simulink model "LKAS"  (R2018b)
settings: Solver=FixedStepDiscrete  StartTime=0.0  StopTime=10.0  FixedStep=0.01  RelTol=1e-3
InitFcn:
  | tmpVer = ver('MATLAB');
  | tmpVer = str2num(tmpVer.Version);
  | % -------------------------------------------------------------------
  | %  MATLAB file generated by Simulink.saveVars on 21-Nov-2019 10:06:14
  | %  MATLAB version: 7.13.0.564 (R2011b)
  | % -------------------------------------------------------------------
  | 
  | 
  | SInt16 = Simulink.AliasType;
  | SInt16.Description = 'Num';
  | if (tmpVer > 7.11)
  | 	SInt16.DataScope = 'Auto';
  | end
  | SInt16.HeaderFile = 'Rte_Type.h';
  | SInt16.BaseType = 'int16';
  | 
  | SInt32 = Simulink.AliasType;
  | SInt32.Description = 'Num';
  | if (tmpVer > 7.11)
  | 	SInt32.DataScope = 'Auto';
  | end
  | SInt32.HeaderFile = 'Rte_Type.h';
  | SInt32.BaseType = 'int32';
  | 
  | SInt8 = Simulink.AliasType;
  | SInt8.Description = 'Num';
  | if (tmpVer > 7.11)
  | 	SInt8.DataScope = 'Auto';
  | end
  | SInt8.HeaderFile = 'Rte_Type.h';
  | SInt8.BaseType = 'int8';
  | 
  | T_A_m2_1024_1_u32 = Simulink.NumericType;
  | T_A_m2_1024_1_u32.Description = 'm2 (square meters  (m2))';
  | if (tmpVer > 7.11)
  | 	T_A_m2_1024_1_u32.DataScope = 'Auto';
  | end
  | T_A_m2_1024_1_u32.HeaderFile = 'Rte_Type.h';
  | T_A_m2_1024_1_u32.DataTypeMode = 'Fixed-point: slope and bias scaling';
  | T_A_m2_1024_1_u32.SignednessBool = false;
  | T_A_m2_1024_1_u32.WordLength = 32;
  | T_A_m2_1024_1_u32.FixedExponent = -10;
  | T_A_m2_1024_1_u32.SlopeAdjustmentFactor = 1;
  | T_A_m2_1024_1_u32.Bias = 0;
  | T_A_m2_1024_1_u32.DataTypeOverride = 'Inherit';
  | T_A_m2_1024_1_u32.IsAlias = true;
  | 
  | T_A_m2_65536_1_u16 = Simulink.NumericType;
  | T_A_m2_65536_1_u16.Description = 'm2 (square meters  (m2))';
  | if (tmpVer > 7.11)
  | 	T_A_m2_65536_1_u16.DataScope = 'Auto';
  | end
  | T_A_m2_65536_1_u16.HeaderFile = 'Rte_Type.h';
  | T_A_m2_65536_1_u16.DataTypeMode = 'Fixed-point: slope and bias scaling';
  | T_A_m2_65536_1_u16.SignednessBool = false;
  | T_A_m2_65536_1_u16.WordLength = 16;
  | T_A_m2_65536_1_u16.FixedExponent = -16;
  | T_A_m2_65536_1_u16.SlopeAdjustmentFactor = 1;
  | T_A_m2_65536_1_u16.Bias = 0;
  | T_A_m2_65536_1_u16.DataTypeOverride = 'Inherit';
  | ... (+4598 lines)
StopFcn:
  | clear  T_A_m2_1024_1_u32 T_A_m2_65536_1_u16 T_A_m2_Float32 T_A_mm2_10_1_u16 T_A_mm2_4_1_s16 T_A_mm2_Float32 T_Cnt_Num_10_1_u32 T_Cnt_Num_1_1_s16 T_Cnt_Num_1_1_s32 T_Cnt_Num_1_1_s8 T_Cnt_Num_1_1_u16 T_Cnt_Num_1_1_u32 T_Cnt_Num_1_1_u8 T_E_J_1_1_s32 T_E_J_Float32 T_E_kJ_128_1_s32 T_E_kJ_Float32 T_E_kwh_10_1_u16 T_E_kwh_Float32 T_Epl_kwhpkm_100_1_u16 T_Epl_kwhpkm_Float32 T_F_N_1_1_s16 T_F_N_Float32 T_I_A_1000_1_u16 T_I_A_1048576_1_s32 T_I_A_2048_1_s16 T_I_A_32_1_s16 T_I_A_Float32 T_I_mA_1_1_s16 T_I_mA_32768_128_s16 T_I_mA_Float32 T_J_kgpm2_128_1_u16 T_J_kgpm2_Float32 T_K_NA_1000_1_s16 T_K_NA_100_1_s16 T_K_NA_100_1_u16 T_K_NA_1024_1_s16 T_K_NA_1024_1_u16 T_K_NA_128_1_s16 T_K_NA_128_1_u16 T_K_NA_128_1_u8 T_K_NA_16777216_1_u32 T_K_NA_16_1_s16 T_K_NA_16_1_u16 T_K_NA_16_1_u8 T_K_NA_1_16_u16 T_K_NA_1_1_s16 T_K_NA_1_1_u16 T_K_NA_1_1_u8 T_K_NA_32768_1_s16 T_K_NA_32768_1_u16 T_K_NA_32_1_s8 T_K_NA_4096_1_u16 T_K_NA_4194304_1_s32 T_K_NA_4194304_1_u16 T_K_NA_65536_1_s32 T_K_NA_65536_1_u16 T_K_NA_8192_1_s16 T_K_NA_8_1_s16 T_K_NA_Float32 T_M_Nm_16_1_s16 T_M_Nm_1_1_s16 T_M_Nm_32768_1_s16 T_M_Nm_32_1_s16 T_M_Nm_4_1_s16 T_M_Nm_512_1_s16 T_M_Nm_Float32 T_P_W_1_4_s16 T_P_W_1_8_s16 T_P_W_Float32 T_P_kW_128_1_s16 T_P_kW_1_8_s16 T_P_kW_8_1_s32 T_P_kW_Float32 T_Pct_pct_1024_1_s32 T_Pct_pct_1024_1_u32 T_Pct_pct_10_1_s16 T_Pct_pct_10_1_u32 T_Pct_pct_128_100_s8 T_Pct_pct_1_1_s16 T_Pct_pct_1_4_u8 T_Pct_pct_255_100_u16 T_Pct_pct_255_100_u8 T_Pct_pct_256_1_s16 T_Pct_pct_256_1_u16 T_Pct_pct_65535_100_u16 T_Pct_pct_Float32 T_R_ohm_1024_1_s16 T_R_ohm_32_1_s16 T_R_ohm_Float32 T_TK_K_16_1_s16 T_TK_K_Float32 T_T_degC_10_400_1_u16 T_T_degC_16_1_s16 T_T_degC_1_40_1_u8 T_T_degC_2_80_1_u8 T_T_degC_Float32 T_U_V_1000_1_u16 T_U_V_10_1_u8 T_U_V_200_1_u8 T_U_V_32_1_s16 T_U_V_4096_1_s16 T_U_V_512_1_s16 T_U_V_65535_8_u16 T_U_V_8192_1_u16 T_U_V_Float32 T_U_mV_1_1_s16 T_U_mV_256_20_u16 T_U_mV_Float32 T_V_l_256_1_s16 T_V_l_4096_1_s16 T_V_l_64_1_s16 T_V_l_65535_100_u16 T_V_l_Float32 T_V_ml_128_1_s16 T_V_ml_1_1_s16 T_V_ml_32768_1_s16 T_V_ml_Float32 T_V_ul_32_1_u16 T_V_ul_Float32 T_Vpl_clpkm_512_1_u16 T_Vpl_clpkm_Float32 T_a_kphps_16_1_s16 T_a_kphps_Float32 T_a_mps2_128_1_s16 T_a_mps2_Float32 T_c_MJpkg_256_1_s16 T_c_MJpkg_Float32 T_c_kJpgpK_1024_1_s16 T_c_kJpgpK_Float32 T_c_kJpkgpK_128_1_u16 T_c_kJpkgpK_Float32 T_chrg_Ah_1_1_s16 T_chrg_Ah_1_1_u16 T_chrg_Ah_1_1_u8 T_chrg_Ah_256_1_u16 T_chrg_Ah_4194304_1_s32 T_chrg_Ah_512_1_u16 T_chrg_Ah_8_1_u16 T_chrg_Ah_Float32 T_cmp_NA_100_1_s16 T_cmp_NA_128_1_s16 T_cmp_NA_16_1_s16 T_cmp_NA_32768_1_u16 T_cmp_NA_Float32 T_d2n_rpmps2_4_1_s16 T_d2n_rpmps2_Float32 T_dPct_pctps_16_1_s16 T_dPct_pctps_256_1_s16 T_dPct_pctps_Float32 T_dT_degCps_128_1_s16 T_dT_degCps_Float32 T_dV_lph_1_1_s16 T_dV_lph_Float32 T_dV_lpm_128_1_s16 T_dV_lpm_32_1_s16 T_dV_lpm_Float32 T_dV_lps_1024_1_u16 T_dV_lps_4_1_u16 T_dV_lps_Float32 T_dV_mlps_1024_1_s16 T_dV_mlps_Float32 T_d_BitField16 T_dm_gps_128_1_s16 T_dm_gps_128_1_u16 T_dm_gps_256_1_u16 T_dm_gps_Float32 T_dm_mgps_1_1_s16 T_dm_mgps_Float32 T_dn_rpmps_1_1_s16 T_dn_rpmps_2_1_s16 T_dn_rpmps_Float32 T_dp_Paps_1_1_s16 T_dp_Paps_Float32 T_dp_kPaps_1_1_s16 T_dp_kPaps_8_1_s16 T_dp_kPaps_Float32 T_dphi_degps_128_1_s16 T_dphi_degps_8_1_s16 T_dphi_degps_Float32 T_dr_ps_256_1_s16 T_dr_ps_Float32 T_drho_mgplps_1_2_s16 T_drho_mgplps_Float32 T_e_NA_1_1_u8 T_f_Hz_1_1_u16 T_f_Hz_1_1_u32 T_f_Hz_64_1_u16 T_f_Hz_8_1_s16 T_f_Hz_Float32 T_g_BitField32 T_l_km_16_1_s16 T_l_km_1_1_u16 T_l_km_1_1_u32 T_l_km_Float32 T_l_m_1024_1_s16 T_l_m_16_1_s16 T_l_m_1_1_u32 T_l_m_Float32 T_l_mm_16_1_s16 T_l_mm_1_1_u16 T_l_mm_4096_1_s16 T_l_mm_4_1_u8 T_l_mm_64_1_s16 T_l_mm_Float32 T_m_g_1_1_s16 T_m_g_2048_1_s16 T_m_g_32_1_u16 T_m_g_Float32 T_m_kg_1024_1_s16 T_m_kg_1_1_s16 T_m_kg_1_1_u32 T_m_kg_Float32 T_m_mg_128_1_s16 T_m_mg_32_1_s16 T_m_mg_Float32 T_n_rpm_1_1_s16 T_n_rpm_1_25_u8 T_n_rpm_256_50_u16 T_n_rpm_2_25_u8 T_n_rpm_4_1_u16 T_n_rpm_Float32 T_p_MPa_64_1_s16 T_p_MPa_Float32 T_p_Pa_1_1_s16 T_p_Pa_Float32 T_p_kPa_1_10_u16 T_p_kPa_1_1_s16 T_p_kPa_1_1_u8 T_p_kPa_256_1_u16 T_p_kPa_32_1_u16 T_p_kPa_64_1_s16 T_p_kPa_Float32 T_phi_deg_100_1_s16 T_phi_deg_1024_1_s16 T_phi_deg_128_1_s16 T_phi_deg_1_1_u8 T_phi_deg_256_1_s16 T_phi_deg_2_1_s8 T_phi_deg_32_1_s16 T_phi_deg_512_6_s32 T_phi_deg_Float32 T_phi_rad_2048_1_s16 T_phi_rad_Float32 T_r_NA_1024_1_s16 T_r_NA_1024_1_u16 T_r_NA_16384_1_s16 T_r_NA_16_1_s16 T_r_NA_256_1_s8 T_r_NA_256_1_u16 T_r_NA_32768_1_u16 T_r_NA_32_1_u16 T_r_NA_4096_1_s16 T_r_NA_65535_2_u16 T_r_NA_8192_1_u16 T_r_NA_Float32 T_rho_gpl_8192_1_s16 T_rho_gpl_Float32 T_rho_kgpm3_16_1_s16 T_rho_kgpm3_Float32 T_rho_mgpl_1_1_s16 T_rho_mgpl_64_1_s16 T_rho_mgpl_Float32 T_t_hour_1_1_s16 T_t_hour_Float32 T_t_m_1_1_u16 T_t_m_Float32 T_t_ms_1_1_s16 T_t_ms_1_1_u16 T_t_ms_1_1_u32 T_t_ms_4096_1_s16 T_t_ms_64_1_s16 T_t_ms_Float32 T_t_s_1000_1_s16 T_t_s_100_1_s16 T_t_s_10_1_s16 T_t_s_10_1_u16 T_t_s_1_1_s16 T_t_s_1_1_u16 T_t_s_1_1_u32 T_t_s_Float32 T_t_us_10_1_u32 T_t_us_1_1_s16 T_t_us_1_1_u32 T_t_us_1_4_u16 T_t_us_Float32 T_v_kph_1_1_u8 T_v_kph_64_1_s16 T_v_kph_64_1_u16 T_v_kph_Float32 T_v_mps_256_1_s16 T_v_mps_Float32 T_w_radps_32_1_s16 T_w_radps_Float32 T_y_BitField8 T_y_BitFieldDiagProgress T_y_BitFieldDiagStatus T_y_NA_1_1_u8 SInt16 SInt32 SInt8 T_BOOLEAN UInt16 UInt32 UInt8 s16 s32 s8 u16 u32 u8
model workspace (MAT data in the model file):
  MCOS : class17 (value not decoded)
  MCOS : class17 (value not decoded)
  MCOS : class17 (value not decoded)
  MCOS : class17 (value not decoded)
  MCOS : class17 (value not decoded)
  MCOS : class17 (value not decoded)
  MCOS : class17 (value not decoded)
  MCOS : class17 (value not decoded)
  MCOS : class17 (value not decoded)
  MCOS : class17 (value not decoded)
  MCOS : class17 (value not decoded)
  MCOS : class17 (value not decoded)
  MCOS : class17 (value not decoded)
  MCOS : class17 (value not decoded)
  MCOS : class17 (value not decoded)
  MCOS : class17 (value not decoded)
  MCOS : class17 (value not decoded)
  MCOS : class17 (value not decoded)
  MCOS : class17 (value not decoded)
  MCOS : class17 (value not decoded)
  MCOS : class17 (value not decoded)
  MCOS : class17 (value not decoded)
  MCOS : class17 (value not decoded)
  MCOS : class17 (value not decoded)
  MCOS : class17 (value not decoded)
  MCOS : class17 (value not decoded)
  MCOS : class17 (value not decoded)
  MCOS : class17 (value not decoded)
  MCOS : class17 (value not decoded)
  MCOS : class17 (value not decoded)
  MCOS : class17 (value not decoded)
  MCOS : class17 (value not decoded)
  MCOS : class17 (value not decoded)
  MCOS : class17 (value not decoded)
  MCOS : class17 (value not decoded)
  MCOS : class17 (value not decoded)
  MCOS : class17 (value not decoded)
  MCOS : class17 (value not decoded)
  MCOS : class17 (value not decoded)
  MCOS : class17 (value not decoded)
  MCOS : class17 (value not decoded)
  MCOS : class17 (value not decoded)
  MCOS : class17 (value not decoded)
  MCOS : class17 (value not decoded)
  MCOS : class17 (value not decoded)
  MCOS : class17 (value not decoded)
  MCOS : class17 (value not decoded)
  MCOS : class17 (value not decoded)
  MCOS : class17 (value not decoded)
  MCOS : class17 (value not decoded)
  MCOS : class17 (value not decoded)
  MCOS : class17 (value not decoded)
  MCOS : class17 (value not decoded)
  MCOS : class17 (value not decoded)
  MCOS : class17 (value not decoded)
  MCOS : class17 (value not decoded)
  MCOS : class17 (value not decoded)
  MCOS : class17 (value not decoded)
  MCOS : class17 (value not decoded)
  MCOS : class17 (value not decoded)
  MCOS : class17 (value not decoded)
  MCOS : class17 (value not decoded)
  MCOS : class17 (value not decoded)
  MCOS : class17 (value not decoded)
  MCOS : class17 (value not decoded)
  MCOS : class17 (value not decoded)
  MCOS : class17 (value not decoded)
  MCOS : class17 (value not decoded)
  MCOS : class17 (value not decoded)
  MCOS : class17 (value not decoded)
  MCOS : class17 (value not decoded)
  MCOS : class17 (value not decoded)
  MCOS : class17 (value not decoded)
  MCOS : class17 (value not decoded)
  MCOS : class17 (value not decoded)
  MCOS : class17 (value not decoded)
  MCOS : class17 (value not decoded)
  MCOS : class17 (value not decoded)
  MCOS : class17 (value not decoded)
  MCOS : class17 (value not decoded)
  MCOS : class17 (value not decoded)
  MCOS : class17 (value not decoded)
  MCOS : class17 (value not decoded)
  MCOS : class17 (value not decoded)
  MCOS : class17 (value not decoded)
  MCOS : class17 (value not decoded)
  MCOS : class17 (value not decoded)
  MCOS : class17 (value not decoded)
  MCOS : class17 (value not decoded)
undefined symbols (not defined in the file): LKA_CarWidth, LKA_SampleTime, LKA_StrRatio_C, LKA_Veh2CamL_C, LKA_Veh2CamW_C, LKA_WhlBaseL_C, LL_CompSWA_C, LL_CrvtPrvwT_C, LL_DesDvt_C, LL_DvtComp_C, LL_DvtPrvwT_C, LL_DvtSpdDet_vDvtSpdMin_C, LL_HdAgExT_C, LL_HdAgPrvwT_C, LL_LAccMax_C, LL_LAccRMax_C, LL_LDW_EarliestWarnLine_C, LL_LDW_LatestWarnLine_C, LL_LDWS_SUPPRESS_HEADING, LL_LFClb_TFC_DiffCtlBalance, LL_LFClb_TFC_DiffCtrlMaxSWA, LL_LFClb_TFC_DiffCtrlRatio, LL_LFClb_TFC_facmGainLutGain1_C, LL_LFClb_TFC_facmGainLutGain2_C, LL_LFClb_TFC_facmIntegRatio, LL_LFClb_TFC_facmKlat_C, LL_LFClb_TFC_FfCtlRatio_C, LL_LFClb_TFC_phiIntegCtlMaxSWA_C, LL_LFClb_TFC_tiKlatPrvwT_C, LL_LFClb_TFC_vGainLutVehSpdLwr_C, LL_LFClb_TFC_vGainLutVehSpdUpr_C, LL_LKA_EarliestWarnLine_C, LL_LKA_LatestWarnLine_C, LL_LKAExPrcs_ExitC0Dvt, LL_LKAExPrcs_ExitC0Swt, LL_LKAExPrcs_tiExitTime1, LL_LKAExPrcs_tiExitTime2, LL_LKAExPrcs_tiExitTime3, LL_LKAS_OUT_OF_CONTROL_LAT_VEL, LL_LKAS_OUT_OF_CONTROL_TTLC, LL_LKASWASyn_M0, LL_LKASWASyn_M1, LL_LKASWASyn_M2, LL_LKASWASyn_M3K, LL_LKASWASyn_SWAaddMax, LL_LKASWASyn_T2, LL_LKASWASyn_tiTrqSwaRtTime, LL_LKASWASyn_tiTrqSwaTime, LL_LKASWASyn_TrqMax, LL_LKASWASyn_TrqSwaAddSwt, LL_LKASWASyn_TrqSwaRateDiff, LL_LSpdCompT_C, LL_lStpLngth_C, LL_MAX_DELAY_EPSSTAR_TIME, LL_MAX_DRIVER_TORQUE_DISABLE, LL_MAX_DRIVER_TORQUE_ENABLE, LL_MAX_LANE_WIDTH_DISABLE, LL_MAX_LANE_WIDTH_ENABLE, LL_MAX_LAT_ACC_DISABLE, LL_MAX_LAT_ACC_ENABLE ... (+29)
libraries: simulink x134, dspstat3 x3, simulink_extras x1
(part 3 of 18)

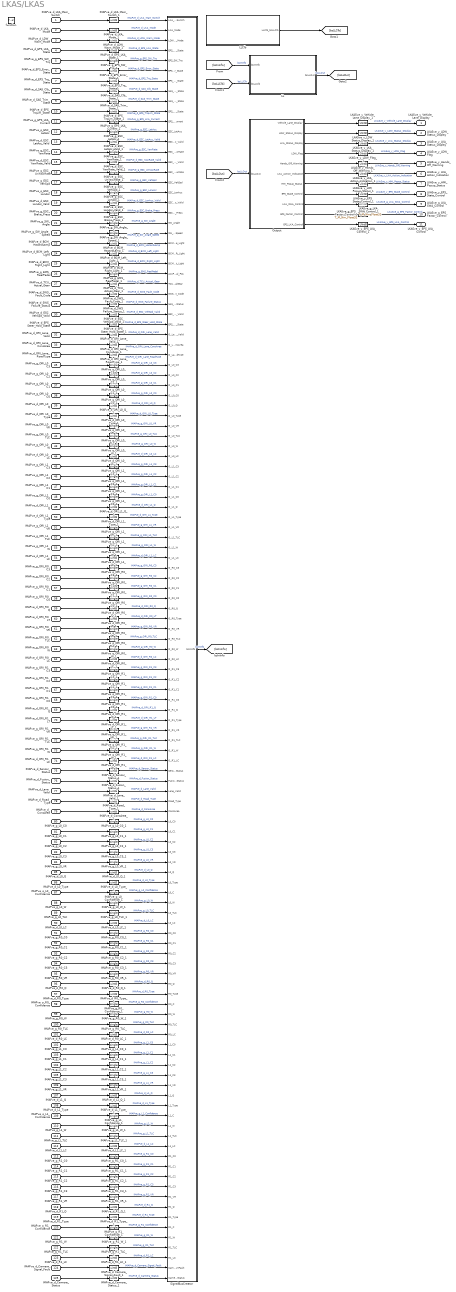
== system LKAS/LKAS ==
  IMAPve_d_LKA_Main_Switch : Inport
  IMAPve_d_LKA_Mode : Inport  Port=2
  IMAPve_d_LDW_Warn_Mode : Inport  Port=3
  IMAPve_d_EPS_LKA_State : Inport  Port=4
  IMAPve_g_EPS_SW_Trq : Inport  Port=5
  IMAPve_d_EPS_Error_State : Inport  Port=6
  IMAPve_d_EPS_Trq_State : Inport  Port=7
  IMAPve_d_SAS_Clb_State : Inport  Port=8
  IMAPve_d_SAS_Trim_State : Inport  Port=9
  IMAPve_d_EPS_TrqLim_State : Inport  Port=10
  IMAPve_g_EPS_LKA_Current : Inport  Port=11
  IMAPve_g_ESC_LatAcc : Inport  Port=12
  IMAPve_d_ESC_LatAcc_Valid : Inport  Port=13
  IMAPve_g_ESC_YawRate : Inport  Port=14
  IMAPve_d_ESC_YawRate_Valid : Inport  Port=15
  IMAPve_g_ESC_UnYawRate : Inport  Port=16
  IMAPve_g_ESC_VehSpd : Inport  Port=17
  IMAPve_g_ESC_LonAcc : Inport  Port=18
  IMAPve_d_ESC_LonAcc_Valid : Inport  Port=19
  IMAPve_g_ESC_Brake_Press : Inport  Port=20
  IMAPve_g_SW_Angle : Inport  Port=21
  IMAPve_g_SW_Angle_Speed : Inport  Port=22
  IMAPve_d_BCM_HazardLamp : Inport  Port=23
  IMAPve_d_BCM_Left_Light : Inport  Port=24
  IMAPve_d_BCM_Right_Light : Inport  Port=25
  IMAPve_g_EMS_RealPedal : Inport  Port=26
  IMAPve_d_TCU_Actual_Gear : Inport  Port=27
  IMAPve_d_SWS_Fault_Code : Inport  Port=28
  IMAPve_d_SWS_Failure_Status : Inport  Port=29
  IMAPve_d_ESC_VehSpd_Valid : Inport  Port=30
  IMAPve_d_EPS_Steer_Hold_State : Inport  Port=31
  IMAPve_d_ORI_Lane_Valid : Inport  Port=32
  IMAPve_d_ORI_Lane_ConsArea : Inport  Port=33
  IMAPve_d_ORI_Lane_RoadType : Inport  Port=34
  IMAPve_g_ORI_L0_C3 : Inport  Port=35
  IMAPve_g_ORI_L0_C2 : Inport  Port=36
  IMAPve_g_ORI_L0_C1 : Inport  Port=37
  IMAPve_g_ORI_L0_C0 : Inport  Port=38
  IMAPve_d_ORI_L0_Q : Inport  Port=39
  IMAPve_d_ORI_L0_Type : Inport  Port=40
  IMAPve_g_ORI_L0_VR : Inport  Port=41
  IMAPve_g_ORI_L0_TLC : Inport  Port=42
  IMAPve_g_ORI_L0_W : Inport  Port=43
  IMAPve_d_ORI_L0_LC : Inport  Port=44
  IMAPve_g_ORI_L1_C3 : Inport  Port=45
  IMAPve_g_ORI_L1_C2 : Inport  Port=46
  IMAPve_g_ORI_L1_C1 : Inport  Port=47
  IMAPve_g_ORI_L1_C0 : Inport  Port=48
  IMAPve_d_ORI_L1_Q : Inport  Port=49
  IMAPve_d_ORI_L1_Type : Inport  Port=50
  IMAPve_g_ORI_L1_VR : Inport  Port=51
  IMAPve_g_ORI_L1_TLC : Inport  Port=52
  IMAPve_g_ORI_L1_W : Inport  Port=53
  IMAPve_d_ORI_L1_LC : Inport  Port=54
  IMAPve_g_ORI_R0_C3 : Inport  Port=55
  IMAPve_g_ORI_R0_C2 : Inport  Port=56
  IMAPve_g_ORI_R0_C1 : Inport  Port=57
  IMAPve_g_ORI_R0_C0 : Inport  Port=58
  IMAPve_d_ORI_R0_Q : Inport  Port=59
  IMAPve_d_ORI_R0_LT : Inport  Port=60
  IMAPve_g_ORI_R0_VR : Inport  Port=61
  IMAPve_g_ORI_R0_TLC : Inport  Port=62
  IMAPve_g_ORI_R0_W : Inport  Port=63
  IMAPve_d_ORI_R0_LC : Inport  Port=64
  IMAPve_g_ORI_R1_C3 : Inport  Port=65
  IMAPve_g_ORI_R1_C2 : Inport  Port=66
  IMAPve_g_ORI_R1_C1 : Inport  Port=67
  IMAPve_g_ORI_R1_C0 : Inport  Port=68
  IMAPve_d_ORI_R1_Q : Inport  Port=69
  IMAPve_d_ORI_R1_LT : Inport  Port=70
  IMAPve_g_ORI_R1_VR : Inport  Port=71
  IMAPve_g_ORI_R1_TLC : Inport  Port=72
  IMAPve_g_ORI_R1_W : Inport  Port=73
  IMAPve_d_ORI_R1_LC : Inport  Port=74
  IMAPve_d_Sensor_Status : Inport  Port=75
  IMAPve_d_Fusion_Status : Inport  Port=76
  IMAPve_d_Lane_Valid : Inport  Port=77
  IMAPve_d_Road_Type : Inport  Port=78
  IMAPve_d_ConsArea : Inport  Port=79
  IMAPve_g_L0_C0 : Inport  Port=80
  IMAPve_g_L0_C1 : Inport  Port=81
  IMAPve_g_L0_C2 : Inport  Port=82
  IMAPve_g_L0_C3 : Inport  Port=83
  IMAPve_g_L0_VR : Inport  Port=84
  IMAPve_d_L0_Q : Inport  Port=85
  IMAPve_d_L0_Type : Inport  Port=86
  IMAPve_g_L0_Confidence : Inport  Port=87
  IMAPve_g_L0_W : Inport  Port=88
  IMAPve_g_L0_TLC : Inport  Port=89
  IMAPve_d_L0_LC : Inport  Port=90
  IMAPve_g_R0_C0 : Inport  Port=91
  IMAPve_g_R0_C1 : Inport  Port=92
  IMAPve_g_R0_C2 : Inport  Port=93
  IMAPve_g_R0_C3 : Inport  Port=94
  IMAPve_g_R0_VR : Inport  Port=95
  IMAPve_d_R0_Q : Inport  Port=96
  IMAPve_d_R0_Type : Inport  Port=97
  IMAPve_g_R0_Confidence : Inport  Port=98
  IMAPve_g_R0_W : Inport  Port=99
  IMAPve_g_R0_TLC : Inport  Port=100
  IMAPve_d_R0_LC : Inport  Port=101
  IMAPve_g_L1_C0 : Inport  Port=102
  IMAPve_g_L1_C1 : Inport  Port=103
  IMAPve_g_L1_C2 : Inport  Port=104
  IMAPve_g_L1_C3 : Inport  Port=105
  IMAPve_g_L1_VR : Inport  Port=106
  IMAPve_d_L1_Q : Inport  Port=107
  IMAPve_d_L1_Type : Inport  Port=108
  IMAPve_g_L1_Confidence : Inport  Port=109
  IMAPve_g_L1_W : Inport  Port=110
  IMAPve_g_L1_TLC : Inport  Port=111
  IMAPve_d_L1_LC : Inport  Port=112
  IMAPve_g_R1_C0 : Inport  Port=113
  IMAPve_g_R1_C1 : Inport  Port=114
  IMAPve_g_R1_C2 : Inport  Port=115
  IMAPve_g_R1_C3 : Inport  Port=116
  IMAPve_g_R1_VR : Inport  Port=117
  IMAPve_d_R1_Q : Inport  Port=118
  IMAPve_d_R1_Type : Inport  Port=119
  IMAPve_g_R1_Confidence : Inport  Port=120
  IMAPve_g_R1_W : Inport  Port=121
  IMAPve_g_R1_TLC : Inport  Port=122
  IMAPve_d_R1_LC : Inport  Port=123
  IMAPve_d_Camera_Signal_Fault : Inport  Port=124
  IMAPve_d_Camera_Status : Inport  Port=125
  function : TriggerPort  TriggerType=function-call  VariantControl=Variant  SampleTimeType=periodic  SampleTime=-1
  IMAPve_d_BCM_HazardLamp_1 : DataTypeConversion  OutDataTypeStr=uint8
  IMAPve_d_BCM_Left_Light_1 : DataTypeConversion  OutDataTypeStr=uint8
  IMAPve_d_BCM_Right_Light_1 : DataTypeConversion  OutDataTypeStr=uint8
  IMAPve_d_Camera_Signal_Fault_1 : DataTypeConversion  OutDataTypeStr=uint8
  IMAPve_d_Camera_Status_1 : DataTypeConversion  OutDataTypeStr=uint8
  IMAPve_d_ConsArea_1 : DataTypeConversion  OutDataTypeStr=uint8
  IMAPve_d_EPS_Error_State_1 : DataTypeConversion  OutDataTypeStr=uint8
  IMAPve_d_EPS_LKA_State_1 : DataTypeConversion  OutDataTypeStr=uint8
  IMAPve_d_EPS_Steer_Hold_State_1 : DataTypeConversion  OutDataTypeStr=uint8
  IMAPve_d_EPS_TrqLim_State_1 : DataTypeConversion  OutDataTypeStr=uint8
  IMAPve_d_EPS_Trq_State_1 : DataTypeConversion  OutDataTypeStr=uint8
  IMAPve_d_ESC_LatAcc_Valid_1 : DataTypeConversion  OutDataTypeStr=uint8
  IMAPve_d_ESC_LonAcc_Valid_1 : DataTypeConversion  OutDataTypeStr=uint8
  IMAPve_d_ESC_VehSpd_Valid_1 : DataTypeConversion  OutDataTypeStr=uint8
  IMAPve_d_ESC_YawRate_Valid_1 : DataTypeConversion  OutDataTypeStr=uint8
  IMAPve_d_Fusion_Status_1 : DataTypeConversion  OutDataTypeStr=uint8
  IMAPve_d_L0_LC_1 : DataTypeConversion  OutDataTypeStr=uint8
  IMAPve_d_L0_Q_1 : DataTypeConversion  OutDataTypeStr=uint8
  IMAPve_d_L0_Type_1 : DataTypeConversion  OutDataTypeStr=uint8
  IMAPve_d_L1_LC_1 : DataTypeConversion  OutDataTypeStr=uint8
  IMAPve_d_L1_Q_1 : DataTypeConversion  OutDataTypeStr=uint8
  IMAPve_d_L1_Type_1 : DataTypeConversion  OutDataTypeStr=uint8
  IMAPve_d_LDW_Warn_Mode_1 : DataTypeConversion  OutDataTypeStr=uint8
  IMAPve_d_LKA_Main_Switch_1 : DataTypeConversion  OutDataTypeStr=uint8
  IMAPve_d_LKA_Mode_1 : DataTypeConversion  OutDataTypeStr=uint8
  IMAPve_d_Lane_Valid_1 : DataTypeConversion  OutDataTypeStr=uint8
  IMAPve_d_ORI_L0_LC_1 : DataTypeConversion  OutDataTypeStr=uint8
  IMAPve_d_ORI_L0_Q_1 : DataTypeConversion  OutDataTypeStr=uint8
  IMAPve_d_ORI_L0_Type_1 : DataTypeConversion  OutDataTypeStr=uint8
  IMAPve_d_ORI_L1_LC_1 : DataTypeConversion  OutDataTypeStr=uint8
  IMAPve_d_ORI_L1_Q_1 : DataTypeConversion  OutDataTypeStr=uint8
  IMAPve_d_ORI_L1_Type_1 : DataTypeConversion  OutDataTypeStr=uint8
  IMAPve_d_ORI_Lane_ConsArea_1 : DataTypeConversion  OutDataTypeStr=uint8
  IMAPve_d_ORI_Lane_RoadType_1 : DataTypeConversion  OutDataTypeStr=uint8
  IMAPve_d_ORI_Lane_Valid_1 : DataTypeConversion  OutDataTypeStr=uint8
  IMAPve_d_ORI_R0_LC_1 : DataTypeConversion  OutDataTypeStr=uint8
  IMAPve_d_ORI_R0_LT_1 : DataTypeConversion  OutDataTypeStr=uint8
  IMAPve_d_ORI_R0_Q_1 : DataTypeConversion  OutDataTypeStr=uint8
  IMAPve_d_ORI_R1_LC_1 : DataTypeConversion  OutDataTypeStr=uint8
  IMAPve_d_ORI_R1_LT_1 : DataTypeConversion  OutDataTypeStr=uint8
  IMAPve_d_ORI_R1_Q_1 : DataTypeConversion  OutDataTypeStr=uint8
  IMAPve_d_R0_LC_1 : DataTypeConversion  OutDataTypeStr=uint8
  IMAPve_d_R0_Q_1 : DataTypeConversion  OutDataTypeStr=uint8
  IMAPve_d_R0_Type_1 : DataTypeConversion  OutDataTypeStr=uint8
  IMAPve_d_R1_LC_1 : DataTypeConversion  OutDataTypeStr=uint8
  IMAPve_d_R1_Q_1 : DataTypeConversion  OutDataTypeStr=uint8
  IMAPve_d_R1_Type_1 : DataTypeConversion  OutDataTypeStr=uint8
  IMAPve_d_Road_Type_1 : DataTypeConversion  OutDataTypeStr=uint8
  IMAPve_d_SAS_Clb_State_1 : DataTypeConversion  OutDataTypeStr=uint8
  IMAPve_d_SAS_Trim_State_1 : DataTypeConversion  OutDataTypeStr=uint8
  IMAPve_d_SWS_Failure_Status_1 : DataTypeConversion  OutDataTypeStr=uint8
  IMAPve_d_SWS_Fault_Code_1 : DataTypeConversion  OutDataTypeStr=uint8
  IMAPve_d_Sensor_Status_1 : DataTypeConversion  OutDataTypeStr=uint8
  IMAPve_d_TCU_Actual_Gear_1 : DataTypeConversion  OutDataTypeStr=uint8
  IMAPve_g_EMS_RealPedal_1 : DataTypeConversion  OutDataTypeStr=single
  IMAPve_g_EPS_LKA_Current_1 : DataTypeConversion  OutDataTypeStr=single
  IMAPve_g_EPS_SW_Trq_1 : DataTypeConversion  OutDataTypeStr=single
  IMAPve_g_ESC_Brake_Press_1 : DataTypeConversion  OutDataTypeStr=single
  IMAPve_g_ESC_LatAcc_1 : DataTypeConversion  OutDataTypeStr=single
  IMAPve_g_ESC_LonAcc_1 : DataTypeConversion  OutDataTypeStr=single
  IMAPve_g_ESC_UnYawRate_1 : DataTypeConversion  OutDataTypeStr=single
  IMAPve_g_ESC_VehSpd_1 : DataTypeConversion  OutDataTypeStr=single
  IMAPve_g_ESC_YawRate_1 : DataTypeConversion  OutDataTypeStr=single
  IMAPve_g_L0_C0_1 : DataTypeConversion  OutDataTypeStr=single
  IMAPve_g_L0_C1_1 : DataTypeConversion  OutDataTypeStr=single
  IMAPve_g_L0_C2_1 : DataTypeConversion  OutDataTypeStr=single
  IMAPve_g_L0_C3_1 : DataTypeConversion  OutDataTypeStr=single
  IMAPve_g_L0_Confidence_1 : DataTypeConversion  OutDataTypeStr=single
  IMAPve_g_L0_TLC_1 : DataTypeConversion  OutDataTypeStr=single
  IMAPve_g_L0_VR_1 : DataTypeConversion  OutDataTypeStr=single
  IMAPve_g_L0_W_1 : DataTypeConversion  OutDataTypeStr=single
  IMAPve_g_L1_C0_1 : DataTypeConversion  OutDataTypeStr=single
  IMAPve_g_L1_C1_1 : DataTypeConversion  OutDataTypeStr=single
  IMAPve_g_L1_C2_1 : DataTypeConversion  OutDataTypeStr=single
  IMAPve_g_L1_C3_1 : DataTypeConversion  OutDataTypeStr=single
  IMAPve_g_L1_Confidence_1 : DataTypeConversion  OutDataTypeStr=single
  IMAPve_g_L1_TLC_1 : DataTypeConversion  OutDataTypeStr=single
  IMAPve_g_L1_VR_1 : DataTypeConversion  OutDataTypeStr=single
  IMAPve_g_L1_W_1 : DataTypeConversion  OutDataTypeStr=single
  IMAPve_g_ORI_L0_C0_1 : DataTypeConversion  OutDataTypeStr=single
  IMAPve_g_ORI_L0_C1_1 : DataTypeConversion  OutDataTypeStr=single
  IMAPve_g_ORI_L0_C2_1 : DataTypeConversion  OutDataTypeStr=single
  IMAPve_g_ORI_L0_C3_1 : DataTypeConversion  OutDataTypeStr=single
  IMAPve_g_ORI_L0_TLC_1 : DataTypeConversion  OutDataTypeStr=single
  IMAPve_g_ORI_L0_VR_1 : DataTypeConversion  OutDataTypeStr=single
  IMAPve_g_ORI_L0_W_1 : DataTypeConversion  OutDataTypeStr=single
  IMAPve_g_ORI_L1_C0_1 : DataTypeConversion  OutDataTypeStr=single
  IMAPve_g_ORI_L1_C1_1 : DataTypeConversion  OutDataTypeStr=single
  IMAPve_g_ORI_L1_C2_1 : DataTypeConversion  OutDataTypeStr=single
  IMAPve_g_ORI_L1_C3_1 : DataTypeConversion  OutDataTypeStr=single
  IMAPve_g_ORI_L1_TLC_1 : DataTypeConversion  OutDataTypeStr=single
  IMAPve_g_ORI_L1_VR_1 : DataTypeConversion  OutDataTypeStr=single
  IMAPve_g_ORI_L1_W_1 : DataTypeConversion  OutDataTypeStr=single
  IMAPve_g_ORI_R0_C0_1 : DataTypeConversion  OutDataTypeStr=single
  IMAPve_g_ORI_R0_C1_1 : DataTypeConversion  OutDataTypeStr=single
  IMAPve_g_ORI_R0_C2_1 : DataTypeConversion  OutDataTypeStr=single
  IMAPve_g_ORI_R0_C3_1 : DataTypeConversion  OutDataTypeStr=single
  IMAPve_g_ORI_R0_TLC_1 : DataTypeConversion  OutDataTypeStr=single
  IMAPve_g_ORI_R0_VR_1 : DataTypeConversion  OutDataTypeStr=single
  IMAPve_g_ORI_R0_W_1 : DataTypeConversion  OutDataTypeStr=single
  IMAPve_g_ORI_R1_C0_1 : DataTypeConversion  OutDataTypeStr=single
  IMAPve_g_ORI_R1_C1_1 : DataTypeConversion  OutDataTypeStr=single
  IMAPve_g_ORI_R1_C2_1 : DataTypeConversion  OutDataTypeStr=single
  IMAPve_g_ORI_R1_C3_1 : DataTypeConversion  OutDataTypeStr=single
  IMAPve_g_ORI_R1_TLC_1 : DataTypeConversion  OutDataTypeStr=single
  IMAPve_g_ORI_R1_VR_1 : DataTypeConversion  OutDataTypeStr=single
  IMAPve_g_ORI_R1_W_1 : DataTypeConversion  OutDataTypeStr=single
  IMAPve_g_R0_C0_1 : DataTypeConversion  OutDataTypeStr=single
  IMAPve_g_R0_C1_1 : DataTypeConversion  OutDataTypeStr=single
  IMAPve_g_R0_C2_1 : DataTypeConversion  OutDataTypeStr=single
  IMAPve_g_R0_C3_1 : DataTypeConversion  OutDataTypeStr=single
  IMAPve_g_R0_Confidence_1 : DataTypeConversion  OutDataTypeStr=single
  IMAPve_g_R0_TLC_1 : DataTypeConversion  OutDataTypeStr=single
  IMAPve_g_R0_VR_1 : DataTypeConversion  OutDataTypeStr=single
  IMAPve_g_R0_W_1 : DataTypeConversion  OutDataTypeStr=single
  IMAPve_g_R1_C0_1 : DataTypeConversion  OutDataTypeStr=single
  IMAPve_g_R1_C1_1 : DataTypeConversion  OutDataTypeStr=single
  IMAPve_g_R1_C2_1 : DataTypeConversion  OutDataTypeStr=single
  IMAPve_g_R1_C3_1 : DataTypeConversion  OutDataTypeStr=single
  IMAPve_g_R1_Confidence_1 : DataTypeConversion  OutDataTypeStr=single
  IMAPve_g_R1_TLC_1 : DataTypeConversion  OutDataTypeStr=single
  IMAPve_g_R1_VR_1 : DataTypeConversion  OutDataTypeStr=single
  IMAPve_g_R1_W_1 : DataTypeConversion  OutDataTypeStr=single
  IMAPve_g_SW_Angle_1 : DataTypeConversion  OutDataTypeStr=single
  IMAPve_g_SW_Angle_Speed_1 : DataTypeConversion  OutDataTypeStr=single
  LKASve_g_EPS_Factor_Control_1 : DataTypeConversion  OutDataTypeStr=T_M_Nm_Float32
  LKASve_g_LKA_SWA_Control_1 : DataTypeConversion  OutDataTypeStr=T_M_Nm_Float32
  LKASve_y_EPS_LKA_Control_1 : DataTypeConversion  OutDataTypeStr=UInt8
  LKASve_y_EPS_State_Control_1 : DataTypeConversion  OutDataTypeStr=UInt8
  LKASve_y_HMI_Popup_Status_1 : DataTypeConversion  OutDataTypeStr=UInt8
  LKASve_y_Hands_Off_Warning_1 : DataTypeConversion  OutDataTypeStr=UInt8
  LKASve_y_LDW_Flag_1 : DataTypeConversion  OutDataTypeStr=UInt8
  LKASve_y_LDW_Status_Display_1 : DataTypeConversion  OutDataTypeStr=UInt8
  LKASve_y_LKA_Action_Indication_1 : DataTypeConversion  OutDataTypeStr=UInt8
  LKASve_y_LKA_Status_Display_1 : DataTypeConversion  OutDataTypeStr=UInt8
  LKASve_y_Vehicle_Lane_Display_1 : DataTypeConversion  OutDataTypeStr=UInt8
  LL : Subsystem
  LLClb : Subsystem
  Output : Subsystem
  SignalBusCreator : Subsystem
  LKASve_y_Vehicle_Lane_Display : Outport
  LKASve_y_LDW_Status_Display : Outport  Port=2
  LKASve_y_LKA_Status_Display : Outport  Port=3
  LKASve_y_LDW_Flag : Outport  Port=4
  LKASve_y_Hands_Off_Warning : Outport  Port=5
  LKASve_y_LKA_Action_Indication : Outport  Port=6
  LKASve_y_HMI_Popup_Status : Outport  Port=7
  LKASve_y_EPS_State_Control : Outport  Port=8
  LKASve_g_LKA_SWA_Control : Outport  Port=9
  LKASve_g_EPS_Factor_Control : Outport  Port=10
  LKASve_y_EPS_LKA_Control : Outport  Port=11
  wires:
  IMAPve_d_LKA_Main_Switch/1 -> IMAPve_d_LKA_Main_Switch_1/1
  IMAPve_d_LKA_Main_Switch_1/1 -> SignalBusCreator/1(LKA_Main_Switch)  "IMAPve_d_LKA_Main_Switch"
  IMAPve_d_LKA_Mode/1 -> IMAPve_d_LKA_Mode_1/1
  IMAPve_d_LKA_Mode_1/1 -> SignalBusCreator/2(LKA_Mode)  "IMAPve_d_LKA_Mode"
  IMAPve_d_LDW_Warn_Mode/1 -> IMAPve_d_LDW_Warn_Mode_1/1
  IMAPve_d_LDW_Warn_Mode_1/1 -> SignalBusCreator/3(LDW_Warn_Mode)  "IMAPve_d_LDW_Warn_Mode"
  IMAPve_d_EPS_LKA_State/1 -> IMAPve_d_EPS_LKA_State_1/1
  IMAPve_d_EPS_LKA_State_1/1 -> SignalBusCreator/4(EPS_LKA_State)  "IMAPve_d_EPS_LKA_State"
  IMAPve_g_EPS_SW_Trq/1 -> IMAPve_g_EPS_SW_Trq_1/1
  IMAPve_g_EPS_SW_Trq_1/1 -> SignalBusCreator/5(EPS_SW_Trq)  "IMAPve_g_EPS_SW_Trq"
  IMAPve_d_EPS_Error_State/1 -> IMAPve_d_EPS_Error_State_1/1
  IMAPve_d_EPS_Error_State_1/1 -> SignalBusCreator/6(EPS_Error_State)  "IMAPve_d_EPS_Error_State"
  IMAPve_d_EPS_Trq_State/1 -> IMAPve_d_EPS_Trq_State_1/1
  IMAPve_d_EPS_Trq_State_1/1 -> SignalBusCreator/7(EPS_Trq_State)  "IMAPve_d_EPS_Trq_State"
  IMAPve_d_SAS_Clb_State/1 -> IMAPve_d_SAS_Clb_State_1/1
  IMAPve_d_SAS_Clb_State_1/1 -> SignalBusCreator/8(SAS_Clb_State)  "IMAPve_d_SAS_Clb_State"
  IMAPve_d_SAS_Trim_State/1 -> IMAPve_d_SAS_Trim_State_1/1
  IMAPve_d_SAS_Trim_State_1/1 -> SignalBusCreator/9(SAS_Trim_State)  "IMAPve_d_SAS_Trim_State"
  IMAPve_d_EPS_TrqLim_State/1 -> IMAPve_d_EPS_TrqLim_State_1/1
  IMAPve_d_EPS_TrqLim_State_1/1 -> SignalBusCreator/10(EPS_TrqLim_State)  "IMAPve_d_EPS_TrqLim_State"
  IMAPve_g_EPS_LKA_Current/1 -> IMAPve_g_EPS_LKA_Current_1/1
  IMAPve_g_EPS_LKA_Current_1/1 -> SignalBusCreator/11(EPS_LKA_Current)  "IMAPve_g_EPS_LKA_Current"
  IMAPve_g_ESC_LatAcc/1 -> IMAPve_g_ESC_LatAcc_1/1
  IMAPve_g_ESC_LatAcc_1/1 -> SignalBusCreator/12(ESC_LatAcc)  "IMAPve_g_ESC_LatAcc"
  IMAPve_d_ESC_LatAcc_Valid/1 -> IMAPve_d_ESC_LatAcc_Valid_1/1
  IMAPve_d_ESC_LatAcc_Valid_1/1 -> SignalBusCreator/13(ESC_LatAcc_Valid)  "IMAPve_d_ESC_LatAcc_Valid"
  IMAPve_g_ESC_YawRate/1 -> IMAPve_g_ESC_YawRate_1/1
  IMAPve_g_ESC_YawRate_1/1 -> SignalBusCreator/14(ESC_YawRate)  "IMAPve_g_ESC_YawRate"
  IMAPve_d_ESC_YawRate_Valid/1 -> IMAPve_d_ESC_YawRate_Valid_1/1
  IMAPve_d_ESC_YawRate_Valid_1/1 -> SignalBusCreator/15(ESC_YawRate_Valid)  "IMAPve_d_ESC_YawRate_Valid"
  IMAPve_g_ESC_UnYawRate/1 -> IMAPve_g_ESC_UnYawRate_1/1
  IMAPve_g_ESC_UnYawRate_1/1 -> SignalBusCreator/16(ESC_UnYawRate)  "IMAPve_g_ESC_UnYawRate"
  IMAPve_g_ESC_VehSpd/1 -> IMAPve_g_ESC_VehSpd_1/1
  IMAPve_g_ESC_VehSpd_1/1 -> SignalBusCreator/17(ESC_VehSpd)  "IMAPve_g_ESC_VehSpd"
  IMAPve_g_ESC_LonAcc/1 -> IMAPve_g_ESC_LonAcc_1/1
  IMAPve_g_ESC_LonAcc_1/1 -> SignalBusCreator/18(ESC_LonAcc)  "IMAPve_g_ESC_LonAcc"
  IMAPve_d_ESC_LonAcc_Valid/1 -> IMAPve_d_ESC_LonAcc_Valid_1/1
  IMAPve_d_ESC_LonAcc_Valid_1/1 -> SignalBusCreator/19(ESC_LonAcc_Valid)  "IMAPve_d_ESC_LonAcc_Valid"
  IMAPve_g_ESC_Brake_Press/1 -> IMAPve_g_ESC_Brake_Press_1/1
  IMAPve_g_ESC_Brake_Press_1/1 -> SignalBusCreator/20(ESC_Brake_Press)  "IMAPve_g_ESC_Brake_Press"
  IMAPve_g_SW_Angle/1 -> IMAPve_g_SW_Angle_1/1
  IMAPve_g_SW_Angle_1/1 -> SignalBusCreator/21(SW_Angle)  "IMAPve_g_SW_Angle"
  IMAPve_g_SW_Angle_Speed/1 -> IMAPve_g_SW_Angle_Speed_1/1
  IMAPve_g_SW_Angle_Speed_1/1 -> SignalBusCreator/22(SW_Angle_Speed)  "IMAPve_g_SW_Angle_Speed"
  IMAPve_d_BCM_HazardLamp/1 -> IMAPve_d_BCM_HazardLamp_1/1
  IMAPve_d_BCM_HazardLamp_1/1 -> SignalBusCreator/23(BCM_Double_Light)  "IMAPve_d_BCM_HazardLamp"
  IMAPve_d_BCM_Left_Light/1 -> IMAPve_d_BCM_Left_Light_1/1
  IMAPve_d_BCM_Left_Light_1/1 -> SignalBusCreator/24(BCM_Left_Light)  "IMAPve_d_BCM_Left_Light"
  IMAPve_d_BCM_Right_Light/1 -> IMAPve_d_BCM_Right_Light_1/1
  IMAPve_d_BCM_Right_Light_1/1 -> SignalBusCreator/25(BCM_Right_Light)  "IMAPve_d_BCM_Right_Light"
  IMAPve_g_EMS_RealPedal/1 -> IMAPve_g_EMS_RealPedal_1/1
  IMAPve_g_EMS_RealPedal_1/1 -> SignalBusCreator/26(AccPedal_Pos)  "IMAPve_g_EMS_RealPedal"
  IMAPve_d_TCU_Actual_Gear/1 -> IMAPve_d_TCU_Actual_Gear_1/1
  IMAPve_d_TCU_Actual_Gear_1/1 -> SignalBusCreator/27(TCU_ActualGear)  "IMAPve_d_TCU_Actual_Gear"
  IMAPve_d_SWS_Fault_Code/1 -> IMAPve_d_SWS_Fault_Code_1/1
  IMAPve_d_SWS_Fault_Code_1/1 -> SignalBusCreator/28(SWS_Fault_Code)  "IMAPve_d_SWS_Fault_Code"
  IMAPve_d_SWS_Failure_Status/1 -> IMAPve_d_SWS_Failure_Status_1/1
  IMAPve_d_SWS_Failure_Status_1/1 -> SignalBusCreator/29(SAS_In_Status)  "IMAPve_d_SWS_Failure_Status"
  IMAPve_d_ESC_VehSpd_Valid/1 -> IMAPve_d_ESC_VehSpd_Valid_1/1
  IMAPve_d_ESC_VehSpd_Valid_1/1 -> SignalBusCreator/30(ESC_VehSpd_Valid)  "IMAPve_d_ESC_VehSpd_Valid"
  IMAPve_d_EPS_Steer_Hold_State/1 -> IMAPve_d_EPS_Steer_Hold_State_1/1
  IMAPve_d_EPS_Steer_Hold_State_1/1 -> SignalBusCreator/31(EPS_SWHold_State)  "IMAPve_d_EPS_Steer_Hold_State"
  IMAPve_d_ORI_Lane_Valid/1 -> IMAPve_d_ORI_Lane_Valid_1/1
  IMAPve_d_ORI_Lane_Valid_1/1 -> SignalBusCreator/32(O_Lane_Valid)  "IMAPve_d_ORI_Lane_Valid"
  IMAPve_d_ORI_Lane_ConsArea/1 -> IMAPve_d_ORI_Lane_ConsArea_1/1
  IMAPve_d_ORI_Lane_ConsArea_1/1 -> SignalBusCreator/33(O_Lane_ConsArea)  "IMAPve_d_ORI_Lane_ConsArea"
  IMAPve_d_ORI_Lane_RoadType/1 -> IMAPve_d_ORI_Lane_RoadType_1/1
  IMAPve_d_ORI_Lane_RoadType_1/1 -> SignalBusCreator/34(O_Lane_RoadType)  "IMAPve_d_ORI_Lane_RoadType"
  IMAPve_g_ORI_L0_C3/1 -> IMAPve_g_ORI_L0_C3_1/1
  IMAPve_g_ORI_L0_C3_1/1 -> SignalBusCreator/35(O_L0_C3)  "IMAPve_g_ORI_L0_C3"
  IMAPve_g_ORI_L0_C2/1 -> IMAPve_g_ORI_L0_C2_1/1
  IMAPve_g_ORI_L0_C2_1/1 -> SignalBusCreator/36(O_L0_C2)  "IMAPve_g_ORI_L0_C2"
  IMAPve_g_ORI_L0_C1/1 -> IMAPve_g_ORI_L0_C1_1/1
  IMAPve_g_ORI_L0_C1_1/1 -> SignalBusCreator/37(O_L0_C1)  "IMAPve_g_ORI_L0_C1"
  IMAPve_g_ORI_L0_C0/1 -> IMAPve_g_ORI_L0_C0_1/1
  IMAPve_g_ORI_L0_C0_1/1 -> SignalBusCreator/38(O_L0_C0)  "IMAPve_g_ORI_L0_C0"
  IMAPve_d_ORI_L0_Q/1 -> IMAPve_d_ORI_L0_Q_1/1
  IMAPve_d_ORI_L0_Q_1/1 -> SignalBusCreator/39(O_L0_Q)  "IMAPve_d_ORI_L0_Q"
  IMAPve_d_ORI_L0_Type/1 -> IMAPve_d_ORI_L0_Type_1/1
  IMAPve_d_ORI_L0_Type_1/1 -> SignalBusCreator/40(O_L0_Type)  "IMAPve_d_ORI_L0_Type"
  IMAPve_g_ORI_L0_VR/1 -> IMAPve_g_ORI_L0_VR_1/1
  IMAPve_g_ORI_L0_VR_1/1 -> SignalBusCreator/41(O_L0_VR)  "IMAPve_g_ORI_L0_VR"
  IMAPve_g_ORI_L0_TLC/1 -> IMAPve_g_ORI_L0_TLC_1/1
  IMAPve_g_ORI_L0_TLC_1/1 -> SignalBusCreator/42(O_L0_TLC)  "IMAPve_g_ORI_L0_TLC"
  IMAPve_g_ORI_L0_W/1 -> IMAPve_g_ORI_L0_W_1/1
  IMAPve_g_ORI_L0_W_1/1 -> SignalBusCreator/43(O_L0_W)  "IMAPve_g_ORI_L0_W"
  IMAPve_d_ORI_L0_LC/1 -> IMAPve_d_ORI_L0_LC_1/1
  IMAPve_d_ORI_L0_LC_1/1 -> SignalBusCreator/44(O_L0_LC)  "IMAPve_d_ORI_L0_LC"
  IMAPve_g_ORI_L1_C3/1 -> IMAPve_g_ORI_L1_C3_1/1
  IMAPve_g_ORI_L1_C3_1/1 -> SignalBusCreator/45(O_L1_C3)  "IMAPve_g_ORI_L1_C3"
  IMAPve_g_ORI_L1_C2/1 -> IMAPve_g_ORI_L1_C2_1/1
  IMAPve_g_ORI_L1_C2_1/1 -> SignalBusCreator/46(O_L1_C2)  "IMAPve_g_ORI_L1_C2"
  IMAPve_g_ORI_L1_C1/1 -> IMAPve_g_ORI_L1_C1_1/1
  IMAPve_g_ORI_L1_C1_1/1 -> SignalBusCreator/47(O_L1_C1)  "IMAPve_g_ORI_L1_C1"
  IMAPve_g_ORI_L1_C0/1 -> IMAPve_g_ORI_L1_C0_1/1
  IMAPve_g_ORI_L1_C0_1/1 -> SignalBusCreator/48(O_L1_C0)  "IMAPve_g_ORI_L1_C0"
  IMAPve_d_ORI_L1_Q/1 -> IMAPve_d_ORI_L1_Q_1/1
  IMAPve_d_ORI_L1_Q_1/1 -> SignalBusCreator/49(O_L1_Q)  "IMAPve_d_ORI_L1_Q"
  IMAPve_d_ORI_L1_Type/1 -> IMAPve_d_ORI_L1_Type_1/1
  IMAPve_d_ORI_L1_Type_1/1 -> SignalBusCreator/50(O_L1_Type)  "IMAPve_d_ORI_L1_Type"
  IMAPve_g_ORI_L1_VR/1 -> IMAPve_g_ORI_L1_VR_1/1
  IMAPve_g_ORI_L1_VR_1/1 -> SignalBusCreator/51(O_L1_VR)  "IMAPve_g_ORI_L1_VR"
  IMAPve_g_ORI_L1_TLC/1 -> IMAPve_g_ORI_L1_TLC_1/1
  IMAPve_g_ORI_L1_TLC_1/1 -> SignalBusCreator/52(O_L1_TLC)  "IMAPve_g_ORI_L1_TLC"
  IMAPve_g_ORI_L1_W/1 -> IMAPve_g_ORI_L1_W_1/1
  IMAPve_g_ORI_L1_W_1/1 -> SignalBusCreator/53(O_L1_W)  "IMAPve_g_ORI_L1_W"
  IMAPve_d_ORI_L1_LC/1 -> IMAPve_d_ORI_L1_LC_1/1
  IMAPve_d_ORI_L1_LC_1/1 -> SignalBusCreator/54(O_L1_LC)  "IMAPve_d_ORI_L1_LC"
  IMAPve_g_ORI_R0_C3/1 -> IMAPve_g_ORI_R0_C3_1/1
  IMAPve_g_ORI_R0_C3_1/1 -> SignalBusCreator/55(O_R0_C3)  "IMAPve_g_ORI_R0_C3"
  IMAPve_g_ORI_R0_C2/1 -> IMAPve_g_ORI_R0_C2_1/1
  IMAPve_g_ORI_R0_C2_1/1 -> SignalBusCreator/56(O_R0_C2)  "IMAPve_g_ORI_R0_C2"
  IMAPve_g_ORI_R0_C1/1 -> IMAPve_g_ORI_R0_C1_1/1
  IMAPve_g_ORI_R0_C1_1/1 -> SignalBusCreator/57(O_R0_C1)  "IMAPve_g_ORI_R0_C1"
  IMAPve_g_ORI_R0_C0/1 -> IMAPve_g_ORI_R0_C0_1/1
  IMAPve_g_ORI_R0_C0_1/1 -> SignalBusCreator/58(O_R0_C0)  "IMAPve_g_ORI_R0_C0"
  IMAPve_d_ORI_R0_Q/1 -> IMAPve_d_ORI_R0_Q_1/1
  IMAPve_d_ORI_R0_Q_1/1 -> SignalBusCreator/59(O_R0_Q)  "IMAPve_d_ORI_R0_Q"
  IMAPve_d_ORI_R0_LT/1 -> IMAPve_d_ORI_R0_LT_1/1
  IMAPve_d_ORI_R0_LT_1/1 -> SignalBusCreator/60(O_R0_Type)  "IMAPve_d_ORI_R0_LT"
  IMAPve_g_ORI_R0_VR/1 -> IMAPve_g_ORI_R0_VR_1/1
  IMAPve_g_ORI_R0_VR_1/1 -> SignalBusCreator/61(O_R0_VR)  "IMAPve_g_ORI_R0_VR"
  IMAPve_g_ORI_R0_TLC/1 -> IMAPve_g_ORI_R0_TLC_1/1
  IMAPve_g_ORI_R0_TLC_1/1 -> SignalBusCreator/62(O_R0_TLC)  "IMAPve_g_ORI_R0_TLC"
  IMAPve_g_ORI_R0_W/1 -> IMAPve_g_ORI_R0_W_1/1
  IMAPve_g_ORI_R0_W_1/1 -> SignalBusCreator/63(O_R0_W)  "IMAPve_g_ORI_R0_W"
  IMAPve_d_ORI_R0_LC/1 -> IMAPve_d_ORI_R0_LC_1/1
  IMAPve_d_ORI_R0_LC_1/1 -> SignalBusCreator/64(O_R0_LC)  "IMAPve_d_ORI_R0_LC"
  IMAPve_g_ORI_R1_C3/1 -> IMAPve_g_ORI_R1_C3_1/1
  IMAPve_g_ORI_R1_C3_1/1 -> SignalBusCreator/65(O_R1_C3)  "IMAPve_g_ORI_R1_C3"
  IMAPve_g_ORI_R1_C2/1 -> IMAPve_g_ORI_R1_C2_1/1
  IMAPve_g_ORI_R1_C2_1/1 -> SignalBusCreator/66(O_R1_C2)  "IMAPve_g_ORI_R1_C2"
  IMAPve_g_ORI_R1_C1/1 -> IMAPve_g_ORI_R1_C1_1/1
  IMAPve_g_ORI_R1_C1_1/1 -> SignalBusCreator/67(O_R1_C1)  "IMAPve_g_ORI_R1_C1"
  IMAPve_g_ORI_R1_C0/1 -> IMAPve_g_ORI_R1_C0_1/1
  IMAPve_g_ORI_R1_C0_1/1 -> SignalBusCreator/68(O_R1_C0)  "IMAPve_g_ORI_R1_C0"
  IMAPve_d_ORI_R1_Q/1 -> IMAPve_d_ORI_R1_Q_1/1
  IMAPve_d_ORI_R1_Q_1/1 -> SignalBusCreator/69(O_R1_Q)  "IMAPve_d_ORI_R1_Q"
  IMAPve_d_ORI_R1_LT/1 -> IMAPve_d_ORI_R1_LT_1/1
  IMAPve_d_ORI_R1_LT_1/1 -> SignalBusCreator/70(O_R1_Type)  "IMAPve_d_ORI_R1_LT"
  IMAPve_g_ORI_R1_VR/1 -> IMAPve_g_ORI_R1_VR_1/1
  IMAPve_g_ORI_R1_VR_1/1 -> SignalBusCreator/71(O_R1_VR)  "IMAPve_g_ORI_R1_VR"
  IMAPve_g_ORI_R1_TLC/1 -> IMAPve_g_ORI_R1_TLC_1/1
  IMAPve_g_ORI_R1_TLC_1/1 -> SignalBusCreator/72(O_R1_TLC)  "IMAPve_g_ORI_R1_TLC"
  IMAPve_g_ORI_R1_W/1 -> IMAPve_g_ORI_R1_W_1/1
  IMAPve_g_ORI_R1_W_1/1 -> SignalBusCreator/73(O_R1_W)  "IMAPve_g_ORI_R1_W"
  IMAPve_d_ORI_R1_LC/1 -> IMAPve_d_ORI_R1_LC_1/1
  IMAPve_d_ORI_R1_LC_1/1 -> SignalBusCreator/74(O_R1_LC)  "IMAPve_d_ORI_R1_LC"
  IMAPve_d_Sensor_Status/1 -> IMAPve_d_Sensor_Status_1/1
  IMAPve_d_Sensor_Status_1/1 -> SignalBusCreator/75(Sensor_Status)  "IMAPve_d_Sensor_Status"
  IMAPve_d_Fusion_Status/1 -> IMAPve_d_Fusion_Status_1/1
  IMAPve_d_Fusion_Status_1/1 -> SignalBusCreator/76(Fusion_Status)  "IMAPve_d_Fusion_Status"
  IMAPve_d_Lane_Valid/1 -> IMAPve_d_Lane_Valid_1/1
  IMAPve_d_Lane_Valid_1/1 -> SignalBusCreator/77(Lane_Valid)  "IMAPve_d_Lane_Valid"
  IMAPve_d_Road_Type/1 -> IMAPve_d_Road_Type_1/1
  IMAPve_d_Road_Type_1/1 -> SignalBusCreator/78(Road_Type)  "IMAPve_d_Road_Type"
  IMAPve_d_ConsArea/1 -> IMAPve_d_ConsArea_1/1
  IMAPve_d_ConsArea_1/1 -> SignalBusCreator/79(ConsArea)  "IMAPve_d_ConsArea"
  IMAPve_g_L0_C0/1 -> IMAPve_g_L0_C0_1/1
  IMAPve_g_L0_C0_1/1 -> SignalBusCreator/80(L0_C0)  "IMAPve_g_L0_C0"
  IMAPve_g_L0_C1/1 -> IMAPve_g_L0_C1_1/1
  IMAPve_g_L0_C1_1/1 -> SignalBusCreator/81(L0_C1)  "IMAPve_g_L0_C1"
  IMAPve_g_L0_C2/1 -> IMAPve_g_L0_C2_1/1
  IMAPve_g_L0_C2_1/1 -> SignalBusCreator/82(L0_C2)  "IMAPve_g_L0_C2"
  IMAPve_g_L0_C3/1 -> IMAPve_g_L0_C3_1/1
  IMAPve_g_L0_C3_1/1 -> SignalBusCreator/83(L0_C3)  "IMAPve_g_L0_C3"
  IMAPve_g_L0_VR/1 -> IMAPve_g_L0_VR_1/1
  IMAPve_g_L0_VR_1/1 -> SignalBusCreator/84(L0_VR)  "IMAPve_g_L0_VR"
  IMAPve_d_L0_Q/1 -> IMAPve_d_L0_Q_1/1
  IMAPve_d_L0_Q_1/1 -> SignalBusCreator/85(L0_Q)  "IMAPve_d_L0_Q"
  IMAPve_d_L0_Type/1 -> IMAPve_d_L0_Type_1/1
  IMAPve_d_L0_Type_1/1 -> SignalBusCreator/86(L0_Type)  "IMAPve_d_L0_Type"
  IMAPve_g_L0_Confidence/1 -> IMAPve_g_L0_Confidence_1/1
  IMAPve_g_L0_Confidence_1/1 -> SignalBusCreator/87(L0_C)  "IMAPve_g_L0_Confidence"
  IMAPve_g_L0_W/1 -> IMAPve_g_L0_W_1/1
  IMAPve_g_L0_W_1/1 -> SignalBusCreator/88(L0_W)  "IMAPve_g_L0_W"
  IMAPve_g_L0_TLC/1 -> IMAPve_g_L0_TLC_1/1
  IMAPve_g_L0_TLC_1/1 -> SignalBusCreator/89(L0_TLC)  "IMAPve_g_L0_TLC"
  IMAPve_d_L0_LC/1 -> IMAPve_d_L0_LC_1/1
  IMAPve_d_L0_LC_1/1 -> SignalBusCreator/90(L0_LC)  "IMAPve_d_L0_LC"
  IMAPve_g_R0_C0/1 -> IMAPve_g_R0_C0_1/1
  IMAPve_g_R0_C0_1/1 -> SignalBusCreator/91(R0_C0)  "IMAPve_g_R0_C0"
  IMAPve_g_R0_C1/1 -> IMAPve_g_R0_C1_1/1
  IMAPve_g_R0_C1_1/1 -> SignalBusCreator/92(R0_C1)  "IMAPve_g_R0_C1"
  IMAPve_g_R0_C2/1 -> IMAPve_g_R0_C2_1/1
  IMAPve_g_R0_C2_1/1 -> SignalBusCreator/93(R0_C2)  "IMAPve_g_R0_C2"
  IMAPve_g_R0_C3/1 -> IMAPve_g_R0_C3_1/1
  IMAPve_g_R0_C3_1/1 -> SignalBusCreator/94(R0_C3)  "IMAPve_g_R0_C3"
  IMAPve_g_R0_VR/1 -> IMAPve_g_R0_VR_1/1
  IMAPve_g_R0_VR_1/1 -> SignalBusCreator/95(R0_VR)  "IMAPve_g_R0_VR"
  IMAPve_d_R0_Q/1 -> IMAPve_d_R0_Q_1/1
  IMAPve_d_R0_Q_1/1 -> SignalBusCreator/96(R0_Q)  "IMAPve_d_R0_Q"
  IMAPve_d_R0_Type/1 -> IMAPve_d_R0_Type_1/1
  IMAPve_d_R0_Type_1/1 -> SignalBusCreator/97(R0_Type)  "IMAPve_d_R0_Type"
  IMAPve_g_R0_Confidence/1 -> IMAPve_g_R0_Confidence_1/1
  IMAPve_g_R0_Confidence_1/1 -> SignalBusCreator/98(R0_C)  "IMAPve_g_R0_Confidence"
  IMAPve_g_R0_W/1 -> IMAPve_g_R0_W_1/1
  IMAPve_g_R0_W_1/1 -> SignalBusCreator/99(R0_W)  "IMAPve_g_R0_W"
  IMAPve_g_R0_TLC/1 -> IMAPve_g_R0_TLC_1/1
  IMAPve_g_R0_TLC_1/1 -> SignalBusCreator/100(R0_TLC)  "IMAPve_g_R0_TLC"
  IMAPve_d_R0_LC/1 -> IMAPve_d_R0_LC_1/1
  IMAPve_d_R0_LC_1/1 -> SignalBusCreator/101(R0_LC)  "IMAPve_d_R0_LC"
  IMAPve_g_L1_C0/1 -> IMAPve_g_L1_C0_1/1
  IMAPve_g_L1_C0_1/1 -> SignalBusCreator/102(L1_C0)  "IMAPve_g_L1_C0"
  IMAPve_g_L1_C1/1 -> IMAPve_g_L1_C1_1/1
  IMAPve_g_L1_C1_1/1 -> SignalBusCreator/103(L1_C1)  "IMAPve_g_L1_C1"
  IMAPve_g_L1_C2/1 -> IMAPve_g_L1_C2_1/1
  IMAPve_g_L1_C2_1/1 -> SignalBusCreator/104(L1_C2)  "IMAPve_g_L1_C2"
  IMAPve_g_L1_C3/1 -> IMAPve_g_L1_C3_1/1
  IMAPve_g_L1_C3_1/1 -> SignalBusCreator/105(L1_C3)  "IMAPve_g_L1_C3"
  IMAPve_g_L1_VR/1 -> IMAPve_g_L1_VR_1/1
  IMAPve_g_L1_VR_1/1 -> SignalBusCreator/106(L1_VR)  "IMAPve_g_L1_VR"
  IMAPve_d_L1_Q/1 -> IMAPve_d_L1_Q_1/1
  IMAPve_d_L1_Q_1/1 -> SignalBusCreator/107(L1_Q)  "IMAPve_d_L1_Q"
  IMAPve_d_L1_Type/1 -> IMAPve_d_L1_Type_1/1
  IMAPve_d_L1_Type_1/1 -> SignalBusCreator/108(L1_Type)  "IMAPve_d_L1_Type"
  IMAPve_g_L1_Confidence/1 -> IMAPve_g_L1_Confidence_1/1
  IMAPve_g_L1_Confidence_1/1 -> SignalBusCreator/109(L1_C)  "IMAPve_g_L1_Confidence"
  IMAPve_g_L1_W/1 -> IMAPve_g_L1_W_1/1
  IMAPve_g_L1_W_1/1 -> SignalBusCreator/110(L1_W)  "IMAPve_g_L1_W"
  IMAPve_g_L1_TLC/1 -> IMAPve_g_L1_TLC_1/1
  IMAPve_g_L1_TLC_1/1 -> SignalBusCreator/111(L1_TLC)  "IMAPve_g_L1_TLC"
  IMAPve_d_L1_LC/1 -> IMAPve_d_L1_LC_1/1
  IMAPve_d_L1_LC_1/1 -> SignalBusCreator/112(L1_LC)  "IMAPve_d_L1_LC"
  IMAPve_g_R1_C0/1 -> IMAPve_g_R1_C0_1/1
  IMAPve_g_R1_C0_1/1 -> SignalBusCreator/113(R1_C0)  "IMAPve_g_R1_C0"
  IMAPve_g_R1_C1/1 -> IMAPve_g_R1_C1_1/1
  IMAPve_g_R1_C1_1/1 -> SignalBusCreator/114(R1_C1)  "IMAPve_g_R1_C1"
  IMAPve_g_R1_C2/1 -> IMAPve_g_R1_C2_1/1
  IMAPve_g_R1_C2_1/1 -> SignalBusCreator/115(R1_C2)  "IMAPve_g_R1_C2"
  IMAPve_g_R1_C3/1 -> IMAPve_g_R1_C3_1/1
  IMAPve_g_R1_C3_1/1 -> SignalBusCreator/116(R1_C3)  "IMAPve_g_R1_C3"
  IMAPve_g_R1_VR/1 -> IMAPve_g_R1_VR_1/1
  IMAPve_g_R1_VR_1/1 -> SignalBusCreator/117(R1_VR)  "IMAPve_g_R1_VR"
  IMAPve_d_R1_Q/1 -> IMAPve_d_R1_Q_1/1
  IMAPve_d_R1_Q_1/1 -> SignalBusCreator/118(R1_Q)  "IMAPve_d_R1_Q"
  IMAPve_d_R1_Type/1 -> IMAPve_d_R1_Type_1/1
  IMAPve_d_R1_Type_1/1 -> SignalBusCreator/119(R1_Type)  "IMAPve_d_R1_Type"
  IMAPve_g_R1_Confidence/1 -> IMAPve_g_R1_Confidence_1/1
  IMAPve_g_R1_Confidence_1/1 -> SignalBusCreator/120(R1_C)  "IMAPve_g_R1_Confidence"
  IMAPve_g_R1_W/1 -> IMAPve_g_R1_W_1/1
  IMAPve_g_R1_W_1/1 -> SignalBusCreator/121(R1_W)  "IMAPve_g_R1_W"
  IMAPve_g_R1_TLC/1 -> IMAPve_g_R1_TLC_1/1
  IMAPve_g_R1_TLC_1/1 -> SignalBusCreator/122(R1_TLC)  "IMAPve_g_R1_TLC"
  IMAPve_d_R1_LC/1 -> IMAPve_d_R1_LC_1/1
  IMAPve_d_R1_LC_1/1 -> SignalBusCreator/123(R1_LC)  "IMAPve_d_R1_LC"
  IMAPve_d_Camera_Signal_Fault/1 -> IMAPve_d_Camera_Signal_Fault_1/1
  IMAPve_d_Camera_Signal_Fault_1/1 -> SignalBusCreator/124(CameraSynFault)  "IMAPve_d_Camera_Signal_Fault"
  IMAPve_d_Camera_Status/1 -> IMAPve_d_Camera_Status_1/1
  IMAPve_d_Camera_Status_1/1 -> SignalBusCreator/125(Camera_Status)  "IMAPve_d_Camera_Status"
  LKASve_y_Vehicle_Lane_Display_1/1 -> LKASve_y_Vehicle_Lane_Display/1  "LKASve_y_Vehicle_Lane_Display"
  Output/1(Vehicle_Lane_Display) -> LKASve_y_Vehicle_Lane_Display_1/1
  LKASve_y_LDW_Status_Display_1/1 -> LKASve_y_LDW_Status_Display/1  "LKASve_y_LDW_Status_Display"
  Output/2(LDW_Status_Display) -> LKASve_y_LDW_Status_Display_1/1
  LKASve_y_LKA_Status_Display_1/1 -> LKASve_y_LKA_Status_Display/1  "LKASve_y_LKA_Status_Display"
  Output/3(LKA_Status_Display) -> LKASve_y_LKA_Status_Display_1/1
  LKASve_y_LDW_Flag_1/1 -> LKASve_y_LDW_Flag/1  "LKASve_y_LDW_Flag"
  Output/4(LDW_Flag) -> LKASve_y_LDW_Flag_1/1
  LKASve_y_Hands_Off_Warning_1/1 -> LKASve_y_Hands_Off_Warning/1  "LKASve_y_Hands_Off_Warning"
  Output/5(Hands_Off_Warning) -> LKASve_y_Hands_Off_Warning_1/1
  LKASve_y_LKA_Action_Indication_1/1 -> LKASve_y_LKA_Action_Indication/1  "LKASve_y_LKA_Action_Indication"
  Output/6(LKA_Action_Indication) -> LKASve_y_LKA_Action_Indication_1/1
  LKASve_y_HMI_Popup_Status_1/1 -> LKASve_y_HMI_Popup_Status/1  "LKASve_y_HMI_Popup_Status"
  Output/7(HMI_Popup_Status) -> LKASve_y_HMI_Popup_Status_1/1
  LKASve_y_EPS_State_Control_1/1 -> LKASve_y_EPS_State_Control/1  "LKASve_y_EPS_State_Control"
  Output/8(EPS_State_Control) -> LKASve_y_EPS_State_Control_1/1
  LKASve_g_LKA_SWA_Control_1/1 -> LKASve_g_LKA_SWA_Control/1  "LKASve_g_LKA_SWA_Control"
  Output/9(LKA_SWA_Control) -> LKASve_g_LKA_SWA_Control_1/1
  LKASve_g_EPS_Factor_Control_1/1 -> LKASve_g_EPS_Factor_Control/1  "LKASve_g_EPS_Factor_Control"
  Output/10(EPS_Factor_Control) -> LKASve_g_EPS_Factor_Control_1/1
  LKASve_y_EPS_LKA_Control_1/1 -> LKASve_y_EPS_LKA_Control/1  "LKASve_y_EPS_LKA_Control"
  Output/11(EPS_LKA_Control) -> LKASve_y_EPS_LKA_Control_1/1
  LL/1(bsLLOut) -> [bsLLOut]  "bsLLOut"
  [bsLLClb] -> LL/2(bsLLClb)  "bsLLClb"
  [bsLLOut] -> Output/1(bsLLOut)  "bsLLOut"
  [bsInInfo] -> LL/1(bsInInfo)  "bsInInfo"
  LLClb/1(LLClb_bsLLClb) -> [bsLLClb]
  SignalBusCreator/1(bsInInfo) -> [bsInInfo]  "bsInInfo"

== system LKAS/LKAS/LL ==
  bsInInfo : Inport
  bsLLClb : Inport  Port=2
  Bus Selector1 : BusSelector  OutputSignals=bsLaneInfo.bsR0Info.R0_Q,bsLaneInfo.bsL0Info.L0_Q
  Bus Selector2 : BusSelector  OutputSignals=bsEPSInfo
  Bus Selector3 : BusSelector  OutputSignals=LKA_State,LDW_State
  Bus Selector4 : BusSelector  OutputSignals=bsLaneInfo.Fusion_AdditionalInf.Carema_Status
  Fault_Diagnostic : Subsystem
  Ground1 : Ground
  Ground3 : Ground
  Human Machine Interface (HMI) : Subsystem
  LL Inputs Mapping : Subsystem
  LL Output (LLOut) : Subsystem
  LLOn : Subsystem
  Subsystem : Subsystem
  Terminator : Terminator
  Version : Constant  Value=200918  OutMin=20410  OutMax=220630  OutDataTypeStr=single
  bsLLOut : Outport
  tag scope: LLMon=global
  wires:
  bsInInfo/1 -> [bsInInfo]
  Ground3/1 -> Human Machine Interface (HMI)/10(HMI_stFaultCSyn)
  Human Machine Interface (HMI)/1(HMI_LDWLKA) -> [HMI_bsLLHMI]  "bsLLHMI"
  [LLOn_bsLDWWarnInfo] -> Human Machine Interface (HMI)/2(HMI_LDWWarn)
  Bus Selector2/1 -> Human Machine Interface (HMI)/7(HMI_EPSInfo)  "<bsEPSInfo>"
  Subsystem/1(On) -> LLOn/Enable
  LL Output (LLOut)/1(LL_bsLLOut) -> bsLLOut/1  "bsLLOut"
  Version/1 -> Terminator/1  "ob_LKA_Version"
  [LLOn_bsLLState] -> Bus Selector3/1
  [bsInInfo] -> LL Inputs Mapping/1(bsInInfo)
  LL Inputs Mapping/1(bsInfo) -> [bsInfo]
  [LLOn_stDACMode] -> Human Machine Interface (HMI)/1(HMI_stDACmode)
  Bus Selector1/2 -> Human Machine Interface (HMI)/6(HMI_L0_Quality)  "<L0_Q>"
  Bus Selector3/1 -> Human Machine Interface (HMI)/3(HMI_LKA_STATE)  "<LKA_State>"
  LLOn/2(LDW_Flag) -> [LLOn_bsLDWWarnInfo]
  Bus Selector1/1 -> Human Machine Interface (HMI)/5(HMI_R0_Quality)  "<R0_Q>"
  [LLOn_bsLLState] -> LL Output (LLOut)/1(LLOut_bsLLState)
  bsLLClb/1 -> [bsLLClb]
  Bus Selector3/2 -> Human Machine Interface (HMI)/4(HMI_LDW_STATE)  "<LDW_State>"
  [LLOn_M] -> LL Output (LLOut)/4(LLOut_M)
  Bus Selector4/1 -> Human Machine Interface (HMI)/9(HMI_Front_Camera_Blocked)  "<Carema_Status>"
  Ground1/1 -> Human Machine Interface (HMI)/8(HMI_camera_common_fault)
  [bsInfo] -> Subsystem/1(bsInfo)
  [bsInfo] -> Bus Selector4/1, Bus Selector2/1, Bus Selector1/1
  [LLOn_phiSWACmd] -> LL Output (LLOut)/2(LLOut_phiSWACmd)
  [HMI_bsLLHMI] -> LL Output (LLOut)/3(LLOut_bsLLHMI)
  Subsystem/2(Mode) -> LLOn/1(stDACMode), [LLOn_stDACMode]
  [bsLLClb] -> LLOn/3(bsLLClb)
  LLOn/1(bsLLState) -> [LLOn_bsLLState]
  LLOn/3(phiSWACmd) -> [LLOn_phiSWACmd]
  [bsSignalFault] -> LLOn/4(bsSignalFault)
  [bsInfo] -> LLOn/2(bsInInfo)
  LLOn/4(M) -> [LLOn_M]
  Fault_Diagnostic/1(bsSignalFault) -> [bsSignalFault]
  [bsInInfo] -> Fault_Diagnostic/1(bsInInfo)
  LLOn/5(LLMon) -> [LLMon]

== system LKAS/LKAS/LLClb ==
  Bus Creator : BusCreator  Inputs=4
  ConstantClb : Subsystem
  LDWClb : Subsystem
  LKAClb : Subsystem
  LLSMConClb : Subsystem
  LLClb_bsLLClb : Outport
  wires:
  ConstantClb/1(ConstantClb) -> Bus Creator/4  "bsConstantClb"
  LLSMConClb/1(LLSMConClb) -> Bus Creator/1  "bsLLSMConClb"
  Bus Creator/1 -> LLClb_bsLLClb/1  "bsLLClb"
  LDWClb/1(LDWClb) -> Bus Creator/2  "bsLDWClb"
  LKAClb/1(LKAClb) -> Bus Creator/3  "bsLKAClb"
